simulink model "lab06"  (R2013a)
settings: Solver=ode45  StartTime=0.0  StopTime=40  RelTol=1e-3  AbsTol=1e-6
values from neighbouring files (symbols this model uses):
  A1 = k1    (= 8)    [FinalLab6.m]    (also in lab6.m = 2)
  a1 = Aw1*sqrt(2*g*h1max)/h1max    [FinalLab6.m]    (also in lab6.m = Aw1*sqrt(2*g*hm1)/hm1)
  A2 = k1    (= 8)    [FinalLab6.m]    (also in lab6.m = 2)
  a2 = Aw2*sqrt(2*g*h2max)/h2max    [FinalLab6.m]    (also in lab6.m = Aw2*sqrt(2*g*hm2)/hm2)
  dfwe = 0.1*fwe1m    [lab6.m]
  dt = 20    [FinalLab6.m]    (also in lab6.m = 10)
  fwe1 = fwe10(i)    [FinalLab6.m]    (also in lab6.m)
  fwe2 = 0.2594    [FinalLab6.m]    (also in lab6.m = 0)
  h10 = (fwe1 / a1) + h20    [FinalLab6.m]    (also in lab6.m = (fwe1+a1*h20)/a1)
  h20 = (fwe1 + fwe2)/a2    [FinalLab6.m]    (also in lab6.m = (fwe2+fwe1)/a2)
settings Model: Creator=LAB320-1552  LastModifiedBy=LAB320-1552
settings DebuggingCC: SolverPrmCheckMsg=none

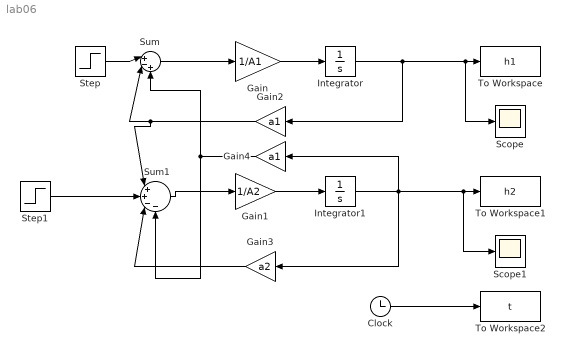
== system lab06 ==
  Clock : Clock
  Gain : Gain  Gain=1/A1
  Gain1 : Gain  Gain=1/A2
  Gain2 : Gain  Gain=a1
  Gain3 : Gain  Gain=a2
  Gain4 : Gain  Gain=a1
  Integrator : Integrator  InitialCondition=h10
  Integrator1 : Integrator  InitialCondition=h20
  Scope : Scope
  Scope1 : Scope
  Step : Step  Time=dt  Before=fwe1  After=fwe1+dfwe  SampleTime=0
  Step1 : Step  Time=dt  Before=fwe2  After=fwe2  SampleTime=0
  Sum : Sum  Inputs=|+-+
  Sum1 : Sum  Inputs=|++--
  To Workspace : ToWorkspace  VariableName=h1  SampleTime=-1
  To Workspace1 : ToWorkspace  VariableName=h2  SampleTime=-1
  To Workspace2 : ToWorkspace  VariableName=t  SampleTime=-1
  wires:
  Step/1 -> Sum/1
  Sum/1 -> Gain/1
  Gain/1 -> Integrator/1
  Integrator/1 -> To Workspace/1, Scope/1, Gain2/1
  Integrator1/1 -> Gain4/1, To Workspace1/1, Scope1/1, Gain3/1
  Clock/1 -> To Workspace2/1
  Gain1/1 -> Integrator1/1
  Sum1/1 -> Gain1/1
  Step1/1 -> Sum1/2
  Gain3/1 -> Sum1/3
  Gain2/1 -> Sum1/1, Sum/2
  Gain4/1 -> Sum1/4, Sum/3
